simulink model "dSpaceLab"  (R2020b)
settings: Solver=VariableStepAuto  StartTime=0.0  StopTime=0.45  RelTol=1e-3
values from neighbouring files (symbols this model uses):
  K_LSF_i = -K_LSF(3)    [dSpaceLab.m]
  K_LSF_p = [K_LSF(2) K_LSF(1)]    [dSpaceLab.m]
  Ke = 6.07/(1560/60*2*pi)    (= 0.037156557868)    [dSpaceLab.m]
  Ki_pi = ki/tau_i    (= 2.51327412287)    [dSpaceLab.m]
  Kp_pi = kp    [dSpaceLab.m]
  Kv_motor = Kv_setup/2    (= 2.02753709245e-06)    [dSpaceLab.m]
  Ra = 1.92/0.83    (= 2.31325301205)    [dSpaceLab.m]
  T_s = 50e-6    (= 5e-05)    [dSpaceLab.m]
  Tf = 0    [dSpaceLab.m]
  V_load = -5    [dSpaceLab.m]
  Vin = 24    [dSpaceLab.m]
libraries: fl_lib x27, nesl_utility x10, ee_lib x1, powerlib_meascontrol x1
settings Model: Creator=sebastian  LastModifiedBy=sebastian

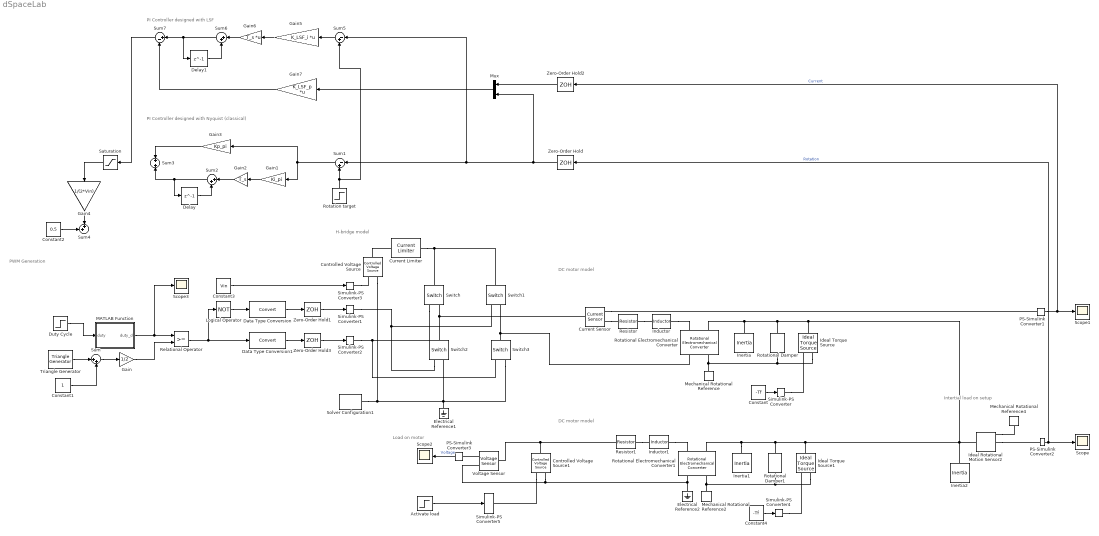
== system dSpaceLab ==
  note: Load on motor
  note: PI Controller designed with Nyquist (classical)
  note: PWM Generation
  note: Intertial load on setup
  note: DC motor model
  note: H-bridge model
  note: DC motor model
  note: PI Controller designed with LSF
  Activate load : Step  Time=2  After=V_load  SampleTime=0
  Constant : Constant  Value=-Tf
  Constant1 : Constant
  Constant2 : Constant  Value=0.5
  Constant3 : Constant  Value=Vin
  Constant4 : Constant  Value=-Tf
  Controlled Voltage Source : fl_lib/Electrical/Electrical Sources/Controlled Voltage Source
  Controlled Voltage Source1 : fl_lib/Electrical/Electrical Sources/Controlled Voltage Source
  Current Limiter : ee_lib/Semiconductors & Converters/Current Limiter  iLim=5 A  vLim=0.1 V  gLim=1e-3 1/Ohm  thermal_mass=100 J/K  initial_temperature=298.15 K
      settings: SourceProductBaseCode=PS  InternalSimscapePortConfiguration="{\"Bottom\":[],\"Left\":[{\"id\":\"p\",\"label\":\"+\",\"type\":\"foundation.electrical.electrical\"}],\"Right\":[{\"id\":\"n\",\"label\":\"-\",\"type\":\"foundation.electrical.electrical\"}],\"Top\":[]}"
  Current Sensor : fl_lib/Electrical/Electrical Sensors/Current Sensor
  Data Type Conversion : DataTypeConversion
  Data Type Conversion1 : DataTypeConversion
  Delay : Delay  DelayLength=1  InitialCondition=0  SampleTime=T_s
  Delay1 : Delay  DelayLength=1  InitialCondition=0  SampleTime=T_s
  Duty Cycle : Step  Time=0  Before=0.5  After=0.72  SampleTime=0
  Electrical Reference1 : fl_lib/Electrical/Electrical Elements/Electrical Reference
  Electrical Reference2 : fl_lib/Electrical/Electrical Elements/Electrical Reference
  Gain : Gain  Gain=1/2
  Gain1 : Gain  Gain=Ki_pi
  Gain2 : Gain  Gain=T_s
  Gain3 : Gain  Gain=Kp_pi
  Gain4 : Gain  Gain=1/(2*Vin)
  Gain5 : Gain  Gain=K_LSF_i  Multiplication=Matrix(K*u)
  Gain6 : Gain  Gain=T_s  Multiplication=Matrix(K*u)
  Gain7 : Gain  Gain=K_LSF_p  Multiplication=Matrix(K*u)
  Ideal Rotational Motion Sensor2 : fl_lib/Mechanical/Mechanical Sensors/Ideal Rotational Motion Sensor  wrap_angle=simscape.enum.onoff.off  offset=0 rad
  Ideal Torque Source : fl_lib/Mechanical/Mechanical Sources/Ideal Torque Source
  Ideal Torque Source1 : fl_lib/Mechanical/Mechanical Sources/Ideal Torque Source
  Inductor : fl_lib/Electrical/Electrical Elements/Inductor  l=La H  r=0 Ohm  g=1e-9 1/Ohm  i_specify=off  i_priority=None  i=0 A  i_nominal_specify=off  i_nominal_unit=A  i_nominal_value=1  v_specify=off  v_priority=None  v=0 V  v_nominal_specify=off  v_nominal_unit=V  v_nominal_value=1  i_L_specify=off  i_L_priority=High  i_L=0 A  i_L_nominal_specify=off  i_L_nominal_unit=A  i_L_nominal_value=1
  Inductor1 : fl_lib/Electrical/Electrical Elements/Inductor  l=La H  r=0 Ohm  g=1e-9 1/Ohm  i_specify=off  i_priority=None  i=0 A  i_nominal_specify=off  i_nominal_unit=A  i_nominal_value=1  v_specify=off  v_priority=None  v=0 V  v_nominal_specify=off  v_nominal_unit=V  v_nominal_value=1  i_L_specify=off  i_L_priority=High  i_L=0 A  i_L_nominal_specify=off  i_L_nominal_unit=A  i_L_nominal_value=1
  Inertia : fl_lib/Mechanical/Rotational Elements/Inertia  inertia=Jr kg*m^2  num_ports=foundation.enum.numPorts2.one  w_specify=off  w_priority=High  w=0 rad/s  w_nominal_specify=off  w_nominal_unit=rad/s  w_nominal_value=1  t_specify=off  t_priority=None  t=0 N*m  t_nominal_specify=off  t_nominal_unit=N*m  t_nominal_value=1
  Inertia1 : fl_lib/Mechanical/Rotational Elements/Inertia  inertia=Jr kg*m^2  num_ports=foundation.enum.numPorts2.one  w_specify=off  w_priority=High  w=0 rad/s  w_nominal_specify=off  w_nominal_unit=rad/s  w_nominal_value=1  t_specify=off  t_priority=None  t=0 N*m  t_nominal_specify=off  t_nominal_unit=N*m  t_nominal_value=1
  Inertia2 : fl_lib/Mechanical/Rotational Elements/Inertia  inertia=JL kg*m^2  num_ports=foundation.enum.numPorts2.one  w_specify=off  w_priority=High  w=0 rad/s  w_nominal_specify=off  w_nominal_unit=rad/s  w_nominal_value=1  t_specify=off  t_priority=None  t=0 N*m  t_nominal_specify=off  t_nominal_unit=N*m  t_nominal_value=1
  Logical Operator : Logic  Operator=NOT  AllPortsSameDT=off  OutDataTypeStr=boolean
  MATLAB Function : MATLAB Function  TreatAsAtomicUnit=on
  Mechanical Rotational Reference : fl_lib/Mechanical/Rotational Elements/Mechanical Rotational Reference
  Mechanical Rotational Reference2 : fl_lib/Mechanical/Rotational Elements/Mechanical Rotational Reference
  Mechanical Rotational Reference4 : fl_lib/Mechanical/Rotational Elements/Mechanical Rotational Reference
  Mux : Mux  Inputs=2
  PS-Simulink Converter1 : nesl_utility/PS-Simulink Converter  PhysicalDomain=network_engine_domain  SubClassName=ps_output  LeftPortType=input  RightPortType=output  PseudoPeriodic=off  Frequencies=[]  Unit=inherit  AffineConversion=off
  PS-Simulink Converter2 : nesl_utility/PS-Simulink Converter  PhysicalDomain=network_engine_domain  SubClassName=ps_output  LeftPortType=input  RightPortType=output  PseudoPeriodic=off  Frequencies=[]  Unit=inherit  AffineConversion=off
  PS-Simulink Converter3 : nesl_utility/PS-Simulink Converter  PhysicalDomain=network_engine_domain  SubClassName=ps_output  LeftPortType=input  RightPortType=output  PseudoPeriodic=off  Frequencies=[]  Unit=inherit  AffineConversion=off
  Relational Operator : RelationalOperator  OutDataTypeStr=boolean  RndMeth=Simplest
  Resistor : fl_lib/Electrical/Electrical Elements/Resistor  R=Ra Ohm  i_specify=off  i_priority=None  i=0 A  i_nominal_specify=off  i_nominal_unit=A  i_nominal_value=1  v_specify=off  v_priority=None  v=0 V  v_nominal_specify=off  v_nominal_unit=V  v_nominal_value=1
  Resistor1 : fl_lib/Electrical/Electrical Elements/Resistor  R=Ra Ohm  i_specify=off  i_priority=None  i=0 A  i_nominal_specify=off  i_nominal_unit=A  i_nominal_value=1  v_specify=off  v_priority=None  v=0 V  v_nominal_specify=off  v_nominal_unit=V  v_nominal_value=1
  Rotation target : Step  After=500/60*2*pi  SampleTime=0
  Rotational Electromechanical Converter : fl_lib/Electrical/Electrical Elements/Rotational Electromechanical Converter  K=Ke V/(rad/s)  i_specify=off  i_priority=None  i=0 A  i_nominal_specify=off  i_nominal_unit=A  i_nominal_value=1  v_specify=off  v_priority=None  v=0 V  v_nominal_specify=off  v_nominal_unit=V  v_nominal_value=1  t_specify=off  t_priority=None  t=0 N*m  t_nominal_specify=off  t_nominal_unit=N*m  t_nominal_value=1  w_specify=off  w_priority=None  w=0 rad/s  w_nominal_specify=off  w_nominal_unit=rad/s  w_nominal_value=1
  Rotational Electromechanical Converter1 : fl_lib/Electrical/Electrical Elements/Rotational Electromechanical Converter  K=Ke V/(rad/s)  i_specify=off  i_priority=None  i=0 A  i_nominal_specify=off  i_nominal_unit=A  i_nominal_value=1  v_specify=off  v_priority=None  v=0 V  v_nominal_specify=off  v_nominal_unit=V  v_nominal_value=1  t_specify=off  t_priority=None  t=0 N*m  t_nominal_specify=off  t_nominal_unit=N*m  t_nominal_value=1  w_specify=off  w_priority=None  w=0 rad/s  w_nominal_specify=off  w_nominal_unit=rad/s  w_nominal_value=1
  Rotational Damper : fl_lib/Mechanical/Rotational Elements/Rotational Damper  D=Kv_motor N*m/(rad/s)  w_specify=off  w_priority=None  w=0 rad/s  w_nominal_specify=off  w_nominal_unit=rad/s  w_nominal_value=1  t_specify=off  t_priority=None  t=0 N*m  t_nominal_specify=off  t_nominal_unit=N*m  t_nominal_value=1
  Rotational Damper1 : fl_lib/Mechanical/Rotational Elements/Rotational Damper  D=Kv_motor N*m/(rad/s)  w_specify=off  w_priority=None  w=0 rad/s  w_nominal_specify=off  w_nominal_unit=rad/s  w_nominal_value=1  t_specify=off  t_priority=None  t=0 N*m  t_nominal_specify=off  t_nominal_unit=N*m  t_nominal_value=1
  Saturation : Saturate  UpperLimit=Vin  LowerLimit=-Vin
  Scope{,1..3} (4 alike) : Scope
  Simulink-PS Converter{,1..5} (6 alike) : nesl_utility/Simulink-PS Converter  PhysicalDomain=network_engine_domain  SubClassName=ps_input  LeftPortType=input  RightPortType=output  PseudoPeriodic=off  Frequencies=[]  NoiseDistribution=none  NoiseParameters=[]  Unit=1  AffineConversion=off  FilteringAndDerivatives=provide  SimscapeFilterOrder=1  InputFilterTimeConstant=0.001  UdotUserProvided=0
  Solver Configuration1 : nesl_utility/Solver Configuration  PhysicalDomain=network_engine_domain  SubClassName=solver  LeftPortType=input  RightPortType=generic  Tones=[]  Harmonics=[]  SimulateNoise=off  Profile=off  UseLocalSampling=off  EnableSwitchedLinearOptims=on  FrequencyDomain=off  UseCCode=off  RelTol=0.001  AbsTol=1e-06  MinStep=1e-09  ToWorkspace=off  RevertToSquareIcSolve=off  NumHomotopyIterations=100  PhasorMode=off  PhasorModeNumHarmonics=1  DoDC=off  ResidualTolerance=1e-09  UseLocalSolver=off  LocalSolverChoice=NE_BACKWARD_EULER_ADVANCER  LocalSolverSampleTime=0.001  DoFixedCost=off  MaxNonlinIter=3  MaxModeIter=2  ComputeImpulses=off  ImpulseIterations=2  LinearAlgebra=auto  EquationFormulation=NE_TIME_EF  DelaysMemoryBudget=1024  AutomaticFiltering=on  FilteringTimeConstant=0.001  PartitionStorageMethod=AS_NEEDED  PartitionMemoryBudget=1024  PartitionMethod=ROBUST
  Sum : Sum  Inputs=|++
  Sum1 : Sum  Inputs=|-+
  Sum2 : Sum  Inputs=|++
  Sum3 : Sum
  Sum4 : Sum  Inputs=++|
  Sum5 : Sum  Inputs=|-+
  Sum6 : Sum  Inputs=|++
  Sum7 : Sum  Inputs=|+-
  Switch{,1..3} (4 alike) : fl_lib/Electrical/Electrical Elements/Switch  R_closed=R_fet Ohm  G_open=G_fet 1/Ohm  Threshold=0.5  i_specify=off  i_priority=None  i=0 A  i_nominal_specify=off  i_nominal_unit=A  i_nominal_value=1  v_specify=off  v_priority=None  v=0 V  v_nominal_specify=off  v_nominal_unit=V  v_nominal_value=1
  Triangle Generator : powerlib_meascontrol/Pulse & Signal Generators/Triangle Generator  Freq=750  Phase=0  Ts=0
  Voltage Sensor : fl_lib/Electrical/Electrical Sensors/Voltage Sensor
  Zero-Order Hold{,1..3} (4 alike) : ZeroOrderHold  SampleTime=T_s
  wires:
  Constant/1 -> Simulink-PS Converter/1
  Triangle Generator/1 -> Sum/1
  Constant1/1 -> Sum/2
  Sum/1 -> Gain/1
  Gain/1 -> Relational Operator/2
  Logical Operator/1 -> Data Type Conversion/1
  Constant3/1 -> Simulink-PS Converter3/1
  PS-Simulink Converter1/1 -> Scope1/1, Zero-Order Hold2/1  "Current"
  Constant4/1 -> Simulink-PS Converter4/1
  PS-Simulink Converter2/1 -> Scope/1, Zero-Order Hold/1  "Rotation"
  Zero-Order Hold/1 -> Mux/2, Sum5/1, Sum1/1
  Rotation target/1 -> Sum5/2, Sum1/2
  Gain1/1 -> Gain2/1
  Gain2/1 -> Sum2/1
  Delay/1 -> Sum2/2
  Sum2/1 -> Sum3/2, Delay/1
  Gain3/1 -> Sum3/1
  Sum1/1 -> Gain1/1, Gain3/1
  Data Type Conversion/1 -> Zero-Order Hold1/1
  Data Type Conversion1/1 -> Zero-Order Hold3/1
  PS-Simulink Converter3/1 -> Scope2/1  "Voltage"
  Saturation/1 -> Gain4/1
  Gain4/1 -> Sum4/2
  Constant2/1 -> Sum4/1
  Activate load/1 -> Simulink-PS Converter5/1
  Sum5/1 -> Gain5/1
  Gain5/1 -> Gain6/1
  Gain6/1 -> Sum6/1
  Delay1/1 -> Sum6/2
  Sum6/1 -> Sum7/1, Delay1/1
  Gain7/1 -> Sum7/2
  Zero-Order Hold2/1 -> Mux/1
  Mux/1 -> Gain7/1
  Relational Operator/1 -> Logical Operator/1, Data Type Conversion1/1
  Zero-Order Hold1/1 -> Simulink-PS Converter1/1
  Zero-Order Hold3/1 -> Simulink-PS Converter2/1
  Sum7/1 -> Saturation/1
  MATLAB Function/1(duty_d) -> Scope3/1, Relational Operator/1
  Duty Cycle/1 -> MATLAB Function/1(duty)
  connections:
  Inductor/RConn1 -- Rotational Electromechanical Converter/LConn1
  Resistor/RConn1 -- Inductor/LConn1
  Rotational Electromechanical Converter/RConn2 -- Ideal Torque Source/RConn2 -- Rotational Damper/RConn1 -- Mechanical Rotational Reference/LConn1
  Simulink-PS Converter/RConn1 -- Ideal Torque Source/RConn1
  Switch1/LConn1 -- Current Limiter/RConn1 -- Switch/LConn1
  Switch2/LConn1 -- Current Sensor/LConn1 -- Switch/RConn2
  Rotational Electromechanical Converter/RConn1 -- Switch3/LConn1 -- Switch1/RConn2
  Simulink-PS Converter1/RConn1 -- Switch2/RConn1 -- Switch1/RConn1
  Simulink-PS Converter2/RConn1 -- Switch/RConn1 -- Switch3/RConn1
  Simulink-PS Converter3/RConn1 -- Controlled Voltage Source/RConn1
  Electrical Reference1/LConn1 -- Controlled Voltage Source/RConn2 -- Solver Configuration1/RConn1 -- Switch2/RConn2 -- Switch3/RConn2
  Current Sensor/RConn2 -- Resistor/LConn1
  Current Sensor/RConn1 -- PS-Simulink Converter1/LConn1
  Mechanical Rotational Reference2/LConn1 -- Ideal Torque Source1/RConn2 -- Rotational Damper1/RConn1 -- Rotational Electromechanical Converter1/RConn2
  Rotational Electromechanical Converter1/RConn1 -- Voltage Sensor/RConn2 -- Controlled Voltage Source1/RConn2 -- Electrical Reference2/LConn1
  Simulink-PS Converter4/RConn1 -- Ideal Torque Source1/RConn1
  Resistor1/LConn1 -- Controlled Voltage Source1/LConn1 -- Voltage Sensor/LConn1
  Inductor1/RConn1 -- Rotational Electromechanical Converter1/LConn1
  Resistor1/RConn1 -- Inductor1/LConn1
  Ideal Rotational Motion Sensor2/RConn1 -- Mechanical Rotational Reference4/LConn1
  Ideal Rotational Motion Sensor2/RConn2 -- PS-Simulink Converter2/LConn1
  Inertia1/LConn1 -- Rotational Electromechanical Converter1/LConn2 -- Rotational Damper1/LConn1 -- Inertia2/LConn1 -- Ideal Rotational Motion Sensor2/LConn1 -- Ideal Torque Source/LConn1 -- Rotational Damper/LConn1 -- Rotational Electromechanical Converter/LConn2 -- Inertia/LConn1 -- Ideal Torque Source1/LConn1
  Voltage Sensor/RConn1 -- PS-Simulink Converter3/LConn1
  Controlled Voltage Source1/RConn1 -- Simulink-PS Converter5/RConn1
  Controlled Voltage Source/LConn1 -- Current Limiter/LConn1

== matlab function dSpaceLab/MATLAB Function ==
  data: duty input; duty_d output
function duty_d = fcn(duty)
    % For discretization of duty cycle steps
    if duty == 0.5
        duty_d = 0.5
    else
        f_sample = 20000;
        f_switch = 750;
        N = 1/(f_sample/f_switch);
        duty_d = N*floor(duty/N);
    end
end
